simulink model "furuta_check"  (R2020a)
settings: Solver=ode45  StartTime=0.0  StopTime=10  RelTol=1e-6  EnableMultiTasking=on
PreLoadFcn:
  | load theta_true
undefined symbols (not defined in the file): DiscIntNeverNeededParam
libraries: vrlib x1
settings Model: Creator=Giampaolo  LastModifiedBy=angelo
settings DataIOCC: LimitDataPoints=on  SaveFormat=Array  ReturnWorkspaceOutputs=off
settings OptimizationCC: ExpressionDepthLimit=2147483647  LifeSpan=inf
settings DebuggingCC: SaveWithParameterizedLinksMsg=none  UnderspecifiedInitializationDetection=Classic  MergeDetectMultiDrivingBlocksExec=none  SolverPrmCheckMsg=warning  FcnCallInpInsideContextMsg=warning  AllowSymbolicDim=off  StateNameClashWarn=warning  SFUnexpectedBacktrackingDiag=warning  SFNoUnconditionalDefaultTransitionDiag=warning  SFExecutionAtInitializationDiag=none  ArithmeticOperatorsInVariantConditions=warning
settings HardwareCC: ProdBitPerPointer=32  ProdBitPerSizeT=32  ProdBitPerPtrDiffT=32  ProdLargestAtomicFloat=None  ProdIntDivRoundTo=Undefined  ProdEndianess=Unspecified  ProdWordSize=32  ProdHWDeviceType=32-bit Generic  TargetHWDeviceType=32-bit Generic
settings ModelReferenceCC: PropagateSignalLabelsOutOfModel=off
settings SFSimCC: SimUseLocalCustomCode=off  CustomCodeUndefinedFunction=UseInterfaceOnly
settings RTWCC: RTWUseLocalCustomCode=off
settings CodeAppCC: StateflowObjectComments=on
settings GRTTargetCC: TargetFcnLib=ansi_tfl_tmw.mat  TargetLangStandard=C89/C90 (ANSI)  CombineOutputUpdateFcns=off  GRTInterface=on
settings ConfigComp: CovMetricSettings=dw  CovHtmlReporting=on  CovSaveCumulativeToWorkspaceVar=on  CovSaveSingleToWorkspaceVar=on  CovExternalEMLEnable=off  CovSFcnEnable=off

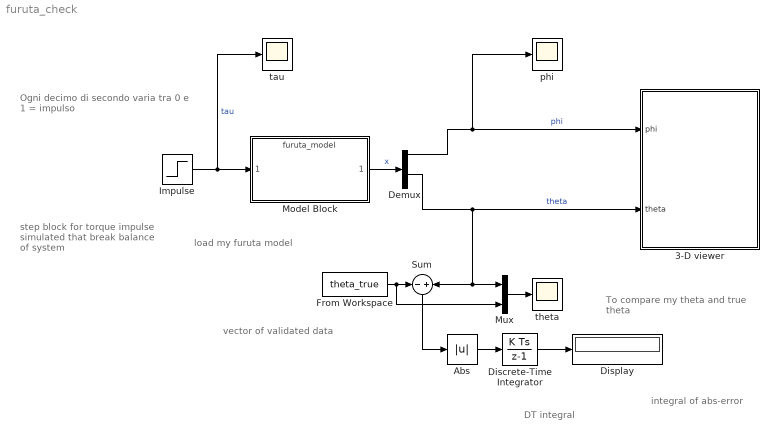
== system furuta_check ==
  note: load my furuta model
  note: To compare my theta and true theta
  note: vector of validated data
  note: step block for torque impulse simulated
      | that break balance of system
  note: DT integral
  note: Ogni decimo di secondo varia tra 0 e 1 = impulso
  note: integral of abs-error
  3-D viewer : Subsystem
  Abs : Abs
  Demux : Demux
  Discrete-Time Integrator : DiscreteIntegrator  SampleTime=0.01  ICPrevOutput=DiscIntNeverNeededParam  ICPrevScaledInput=DiscIntNeverNeededParam
  Display : Display
  From Workspace : FromWorkspace  VariableName=theta_true  SampleTime=0.01  Interpolate=off  OutputAfterFinalValue=Holding final value
  Impulse : Step  Time=0.1  Before=1  After=0  SampleTime=0
  Model Block : ModelReference  ModelNameDialog=furuta_model.slx  SimulationMode=Normal  ModelReferenceVersion=1.14
  Mux : Mux  Inputs=2
  Sum : Sum  Inputs=-+
  phi : Scope
  tau : Scope
  theta : Scope
  wires:
  Demux/3 -> 3-D viewer/2(theta), Mux/1, Sum/2  "theta"
  Demux/1 -> 3-D viewer/1(phi), phi/1  "phi"
  Impulse/1 -> Model Block/1, tau/1  "tau"
  Model Block/1 -> Demux/1  "x"
  From Workspace/1 -> Mux/2, Sum/1
  Sum/1 -> Abs/1
  Discrete-Time Integrator/1 -> Display/1
  Abs/1 -> Discrete-Time Integrator/1
  Mux/1 -> theta/1

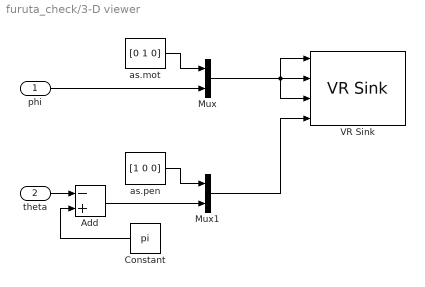
== system furuta_check/3-D viewer ==
  phi : Inport
  theta : Inport  Port=2
  Add : Sum  Inputs=-+
  Constant : Constant  Value=pi
  Mux : Mux  Inputs=2
  Mux1 : Mux  Inputs=2
  VR Sink : vrlib/VR Sink  InstantiateOnLoad=on  SampleTime=0.03  ViewEnable=on  RemoteChange=off  RemoteView=on  FieldsWritten=Puleggia_8.rotation.4.1.1.double#Puleggia.rotation.4.1.1.double#LinkP-L.rotation.4.1.1.double#pispolo.rotation.4.1.1.double  WorldFileName=fu.wrl  AutoView=off  VideoDimensions=[]  AllowVariableSize=off
  as.mot : Constant  Value=[0 1 0]
  as.pen : Constant  Value=[1 0 0]
  wires:
  as.mot/1 -> Mux/1
  as.pen/1 -> Mux1/1
  Mux/1 -> VR Sink/1, VR Sink/3, VR Sink/2
  Mux1/1 -> VR Sink/4
  Add/1 -> Mux1/2
  Constant/1 -> Add/2
  phi/1 -> Mux/2
  theta/1 -> Add/1
